simulink model "lqr_int"  (R2023b)
settings: Solver=FixedStepAuto  StartTime=0.0  StopTime=SIMTIME  FixedStep=SIMSTEP  RelTol=1e-3
undefined symbols (not defined in the file): A, B, bias, Bv, C, Ki, Klqr, ref, wave_ampl, wave_length, x0, x0int
settings Model: Creator=X20  LastModifiedBy=Lorenzo-Desk
settings DataIOCC: ReturnWorkspaceOutputs=off

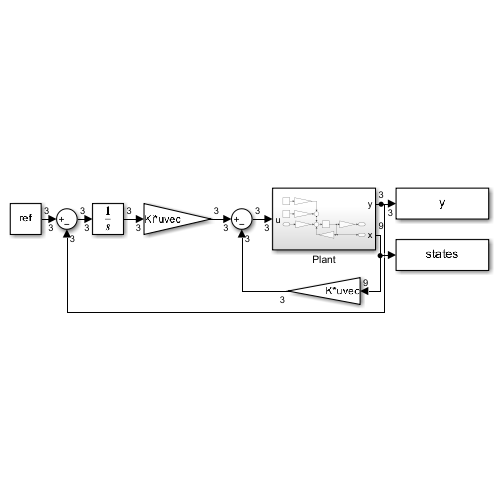
[thumbnail: Simulink's stored preview of the top-level diagram]
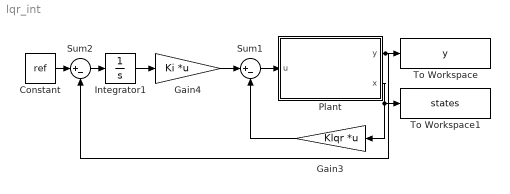
== system lqr_int ==
  Constant : Constant  Value=ref
  Gain3 : Gain  Gain=Klqr  Multiplication=Matrix(K*u) (u vector)
  Gain4 : Gain  Gain=Ki  Multiplication=Matrix(K*u) (u vector)
  Integrator1 : Integrator  InitialCondition=x0int
  Plant : Subsystem
  Sum1 : Sum  Inputs=|+-
  Sum2 : Sum  Inputs=|+-
  To Workspace : ToWorkspace  VariableName=y  SaveFormat=Timeseries  SampleTime=-1
  To Workspace1 : ToWorkspace  VariableName=states  SaveFormat=Timeseries  SampleTime=-1
  wires:
  Gain3/1 -> Sum1/2
  Gain4/1 -> Sum1/1
  Integrator1/1 -> Gain4/1
  Sum2/1 -> Integrator1/1
  Constant/1 -> Sum2/1
  Sum1/1 -> Plant/1(u)
  Plant/2(x) -> Gain3/1, To Workspace1/1
  Plant/1(y) -> Sum2/2, To Workspace/1

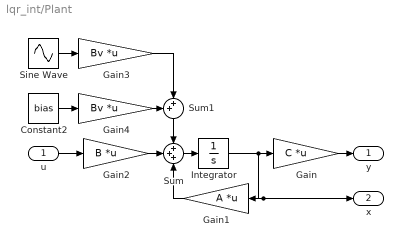
== system lqr_int/Plant ==
  u : Inport
  Constant2 : Constant  Value=bias
  Gain : Gain  Gain=C  Multiplication=Matrix(K*u) (u vector)
  Gain1 : Gain  Gain=A  Multiplication=Matrix(K*u) (u vector)
  Gain2 : Gain  Gain=B  Multiplication=Matrix(K*u) (u vector)
  Gain3 : Gain  Gain=Bv  Multiplication=Matrix(K*u) (u vector)
  Gain4 : Gain  Gain=Bv  Multiplication=Matrix(K*u) (u vector)
  Integrator : Integrator  InitialCondition=x0
  Sine Wave : Sin  Amplitude=wave_ampl  Frequency=1./wave_length  SampleTime=0
  Sum : Sum  Inputs=+++
  Sum1 : Sum  Inputs=++|
  y : Outport
  x : Outport  Port=2
  wires:
  Gain/1 -> y/1
  u/1 -> Gain2/1
  Sum/1 -> Integrator/1
  Integrator/1 -> x/1, Gain1/1, Gain/1
  Gain1/1 -> Sum/3
  Gain2/1 -> Sum/2
  Sum1/1 -> Sum/1
  Gain4/1 -> Sum1/1
  Constant2/1 -> Gain4/1
  Sine Wave/1 -> Gain3/1
  Gain3/1 -> Sum1/2
